simulink model "CH9_1_firstEV_00"  (R2022a)
settings: Solver=VariableStepAuto  StartTime=0.0  StopTime=200  RelTol=1e-3
values from neighbouring files (symbols this model uses):
  Batt_R0 = 0.05    [CH9_1_firstEV_00Param.m]    (also in CH9_1_firstEV_01Param.m; CH9_1_firstEV_02Param.m)
  Motor_kTorque = 0.01    [CH9_1_firstEV_00Param.m]    (also in CH9_1_firstEV_01Param.m; CH9_1_firstEV_02Param.m)
  Motor_TrqKi = 400    [CH9_1_firstEV_00Param.m]    (also in CH9_1_firstEV_01Param.m; CH9_1_firstEV_02Param.m)
  Motor_TrqKp = 600    [CH9_1_firstEV_00Param.m]    (also in CH9_1_firstEV_01Param.m; CH9_1_firstEV_02Param.m)
  Motor_TrqMax = 400    [CH9_1_firstEV_00Param.m]    (also in CH9_1_firstEV_01Param.m; CH9_1_firstEV_02Param.m)
  Motor_TrqMin = -400    [CH9_1_firstEV_00Param.m]    (also in CH9_1_firstEV_01Param.m; CH9_1_firstEV_02Param.m)
  Motor_tTorque = 0.02    [CH9_1_firstEV_00Param.m]    (also in CH9_1_firstEV_01Param.m; CH9_1_firstEV_02Param.m)
  VehMass = 1200    [CH9_1_firstEV_00Param.m]    (also in CH9_1_firstEV_01Param.m)
libraries: fl_lib x34, nesl_utility x9, sdl_lib x6, autolibshared x1, ee_lib x1, slpidlib x1
settings Model: Creator=amyyang  LastModifiedBy=amyyang
settings SolverCC: ZeroCrossAlgorithm=Adaptive  AlgebraicLoopSolver=TrustRegion
settings DataIOCC: ReturnWorkspaceOutputs=off
settings DebuggingCC: IgnoredZcDiagnostic=none  UnconnectedInputMsg=warning  UnconnectedOutputMsg=warning  UnconnectedLineMsg=warning  SFMachineParentedDataDiag=warning  ArithmeticOperatorsInVariantConditions=warning
settings SFSimCC: SimUseLocalCustomCode=off  CustomCodeUndefinedFunction=UseInterfaceOnly
settings RTWCC: RTWUseLocalCustomCode=off  DLArmComputeVersion=19.05
settings SimscapeCC: SimscapeLogType=local  SimscapeLogSimulationStatistics=on  SimscapeLogToSDI=on  SimscapeLogLimitData=off

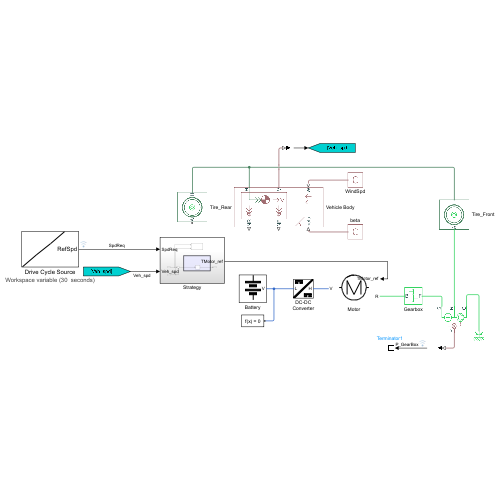
[thumbnail: Simulink's stored preview of the top-level diagram]
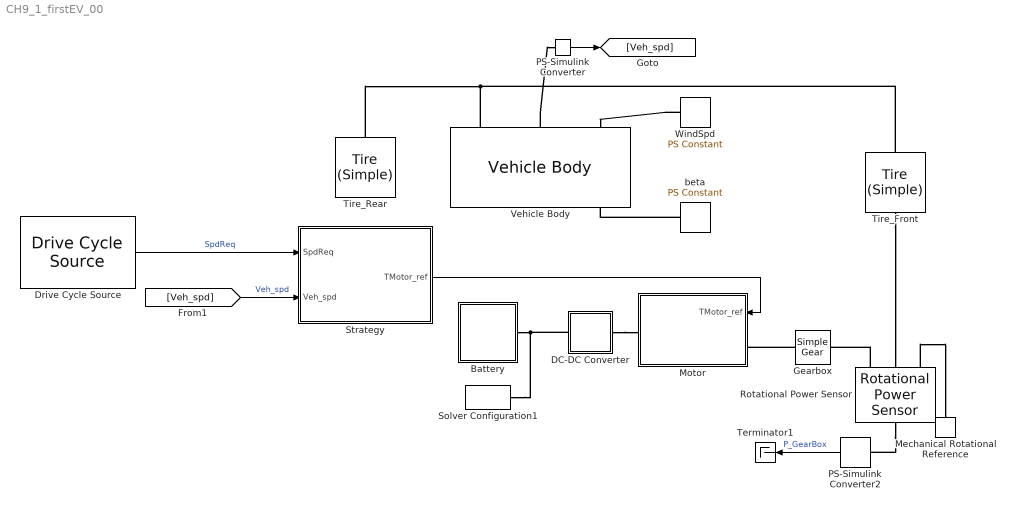
== system CH9_1_firstEV_00 ==
  Battery : Subsystem
      mask Display:
      | % Plot points to set plot range
      | color('white');plot(1.5, 2.5);plot(-1.5, -2)
      | color('black');
      | % Battery icon
      | plot([0 0], [2.5 1.3])
      | plot([0 0], [-0.6 -1.6])
      | patch([-1 1 1 -1]*0.4, [1 1 -1 -1]*0.15+0.7,[0;0;0]);
      | patch([-1 1 1 -1]*0.4, [1 1 -1 -1]*0.15-0.6,[0;0;0]);
      | patch([-1 1 1 -1]*0.8, [1 1 -1 -1]*0.15+1.3,[0;0;0]);
      | patch([-1 1 1 -1]*0.8, [1 1 -1 -1]*0.15+0.0,[0;0;0]);
  DC-DC Converter : Subsystem
      mask Display:
      | patch([-0.9 -1 -1 0.9 1 1 -0.9],[-1 -1 -0.9 1 1 0.9 -1],[0 0 0])
      | 
      | patch([-0.8 -0.1 -0.1 -0.8],[0.85 0.85 0.75 0.75],[0 0 0])
      | patch([-0.8 -0.55 -0.55 -0.8],[0.65 0.65 0.55 0.55],[0 0 0])
      | patch([-0.35 -0.1 -0.1 -0.35],[0.65 0.65 0.55 0.55],[0 0 0])
      | 
      | patch([-0.8 -0.1 -0.1 -0.8]*-1,[0.65 0.65 0.55 0.55]*-1,[0 0 0])
      | patch([-0.8 -0.55 -0.55 -0.8]*-1,[0.85 0.85 0.75 0.75]*-1,[0 0 0])
      | patch([-0.35 -0.1 -0.1 -0.35]*-1,[0.85 0.85 0.75 0.75]*-1,[0 0 0])
  Drive Cycle Source : autolibshared/Drive Cycle Source  cycleVar=Workspace variable  wsVar=myCycleS  fileVar=cycleFTP75.mat  tfinal="30  seconds"  cycleRepeat=off  outAccPort=off  outGearPort=off  gearList=No gear data  t_wot1=5  xdot_woto=0  xdot_wot1=30  t_wot2=20  xdot_wot2=0  t_wotend=30  srcUnit=m/s  outUnit=m/s  srcAccUnit=m/s/s  outAccUnit=m/s^2  dt=0  aMode=1  faultOption=off  velBnd=2  velBndUnit=mph  inUnit=m/s  timeBnd=1  failOption=off  stopSim=off  maxFaultCnt=10  maxFaultTime=2  maxTotFaultTime=15  traceOption=off  dtTrace=1  traceWindow=10  lastDCname=Custom Data Set  lastOutUnit=mph  lastDT=0  lastTB=1  lastSB=2  forceCalcBound=off
      settings: SourceProductBaseCode=PW,DR,MT,VE
  Gearbox : sdl_lib/Gears/Simple Gear  ratio=Motor_GearRio  rotation_direction=sdl.enum.shaftOutputDirection.same  friction_model=sdl.enum.gear_efficiencies_load.constant  T_noload=0.1 N*m  T_nom=5 N*m  efficiency_nom=0.8  efficiency=Motor_GearEff  temperature_TLU=[ 280 300 320 ] K  load_TLU=[ 1 5 10 ] N*m  efficiency_TLU=[ 0.95 0.9 0.85 ]  efficiency_TLU2=[ 0.85 0.8 0.75; 0.95 0.9 0.85; 0.85 0.8 0.7 ]  w_thr=0.01 rad/s  pwr_thr=0.001 W  backlash_model=sdl.enum.backlashModel.Off  backlash_distance=1e-3 mm  x0=0 mm  r_base=0.1 m  hardstop_model=simscape.enum.hardstop.smooth  transition=1e-4 mm  backlash_stiffness=1e7 N/m  backlash_damping=1e6 N*s/m  e=0  v_tol=0.001 m/s  mu_visc=[ 0 0 ] N*m/(rad/s)  enable_faults=simscape.enum.onoff.off  efficiency_fault=0.05  external_fault=simscape.enum.onoff.off  temporal_fault=simscape.enum.onoff.off  fault_time=5 s  fault_angles=pi / 12 rad  report_fault=simscape.enum.assert.action.none  thermal_mass=50 J/K  temperature_specify=off  temperature_priority=High  temperature=300 K  temperature_nominal_specify=off  temperature_nominal_unit=K  temperature_nominal_value=1  x_backlash_specify=off  x_backlash_priority=None  x_backlash=0 mm  x_backlash_nominal_specify=off  x_backlash_nominal_unit=mm  x_backlash_nominal_value=1  f_hardstop_specify=off  f_hardstop_priority=None  f_hardstop=0 N  f_hardstop_nominal_specify=off  f_hardstop_nominal_unit=N  f_hardstop_nominal_value=1  v_backlash_specify=off  v_backlash_priority=None  v_backlash=0 m/s  v_backlash_nominal_specify=off  v_backlash_nominal_unit=m/s  v_backlash_nominal_value=1
      settings: SourceProductName=Driveline  LogSimulationData=on
  Mechanical Rotational Reference : fl_lib/Mechanical/Rotational Elements/Mechanical Rotational Reference
      settings: SourceProductBaseCode=PW,SS,VE
  Motor : Subsystem
      mask Display:
      | % Circle
      | plot(sin(0:0.1:2.2*pi)*0.9,cos(0:0.1:2.2*pi)*0.9);
      | 
      | % In/out
      | plot([-1.1 -0.9],[0 0]);
      | plot([1.1 0.9],[0 0]);
      | 
      | % 'M'
      | plot([0.5 0.5],[-0.5 0.5]);
      | plot([-0.5 -0.5],[-0.5 0.5]);
      | plot([0.5 0],[0.5 -0.5]);
      | plot([-0.5 0],[0.5 -0.5]);
      | 
      | % Plot points to set plot range
      | color('white');plot(1.9,1.2);plot(-1.9,-1.2)
      | color('black');
  PS-Simulink Converter : nesl_utility/PS-Simulink Converter  PhysicalDomain=network_engine_domain  SubClassName=ps_output  LeftPortType=input  RightPortType=output  PseudoPeriodic=off  Frequencies=[]  VectorFormat=1-D array  Unit=m/s  AffineConversion=off
      settings: SourceProductBaseCode=SS,PW,VE
  PS-Simulink Converter2 : nesl_utility/PS-Simulink Converter  PhysicalDomain=network_engine_domain  SubClassName=ps_output  LeftPortType=input  RightPortType=output  PseudoPeriodic=off  Frequencies=[]  VectorFormat=1-D array  Unit=kW  AffineConversion=off
      settings: SourceProductName=Utilities
  Rotational Power Sensor : sdl_lib/Sensors/Rotational Power Sensor  measurement_type=1  averaging_period=1 s  max_frequency=1000 Hz  max_speed=1000 rpm
      settings: SourceProductBaseCode=LD  InternalSimscapePortConfiguration="{\"Bottom\":[],\"Left\":[{\"id\":\"S\",\"label\":\"S\",\"type\":\"foundation.mechanical.rotational.rotational\"},{\"id\":\"R\",\"label\":\"R\",\"type\":\"foundation.mechanical.rotational.rotational\"},{\"id\":\"C\",\"label\":\"C\",\"type\":\"foundation.mechanical.rotational.rotational\"}],\"Right\":[{\"id\":\"P\",\"label\":\"P\",\"type\":\"output\"}],\"Top\":[]}"
  Solver Configuration1 : nesl_utility/Solver Configuration  PhysicalDomain=network_engine_domain  SubClassName=solver  LeftPortType=input  RightPortType=generic  Tones=[]  Harmonics=[]  SimulateNoise=off  Profile=off  UseLocalSampling=off  EnableSwitchedLinearOptims=on  FrequencyDomain=off  UseCCode=off  RelTol=0.001  AbsTol=1e-06  MinStep=1e-09  ToWorkspace=off  RevertToSquareIcSolve=off  NumHomotopyIterations=100  PhasorMode=off  PhasorModeNumHarmonics=1  IndexReductionMethod=DerivativeReplacement  DoDC=off  ResidualTolerance=1e-9  UseLocalSolver=off  LocalSolverChoice=NE_PARTITIONING_ADVANCER  LocalSolverSampleTime=0.005  DoFixedCost=off  MaxNonlinIter=5  MaxModeIter=2  ComputeImpulses=off  ImpulseIterations=2  LinearAlgebra=auto  LinearAlgebraNumThread=0  EquationFormulation=NE_TIME_EF  DelaysMemoryBudget=1024  AutomaticFiltering=on  FilteringTimeConstant=0.001  PartitionStorageMethod=EXHAUSTIVE  PartitionMemoryBudget=1024  PartitionMethod=ROBUST
      settings: SourceProductName=Utilities
  Strategy : Subsystem
  Terminator1 : Terminator
  Tire_Front : sdl_lib/Tires & Vehicles/Tire (Simple)  r_tire=Tire_R m  model_compliance=0  stiffness=Tire_K N/m  damping=Tire_Damp N/(m/s)  model_inertia=0  tire_inertia=Tire_Inertia kg*m^2  initial_velocity=Tire_IniSpd rad/s
      settings: SourceProductBaseCode=LD  LogSimulationData=on  InternalSimscapePortConfiguration="{\"Bottom\":[],\"Left\":[{\"id\":\"A\",\"label\":\"A\",\"type\":\"foundation.mechanical.rotational.rotational\"}],\"Right\":[{\"id\":\"H\",\"label\":\"H\",\"type\":\"foundation.mechanical.translational.translational\"}],\"Top\":[]}"
  Tire_Rear : sdl_lib/Tires & Vehicles/Tire (Simple)  r_tire=Tire_R m  model_compliance=0  stiffness=Tire_K N/m  damping=Tire_Damp N/(m/s)  model_inertia=0  tire_inertia=Tire_Inertia kg*m^2  initial_velocity=Tire_IniSpd rad/s
      settings: SourceProductBaseCode=LD  LogSimulationData=on  InternalSimscapePortConfiguration="{\"Bottom\":[],\"Left\":[{\"id\":\"A\",\"label\":\"A\",\"type\":\"foundation.mechanical.rotational.rotational\"}],\"Right\":[{\"id\":\"H\",\"label\":\"H\",\"type\":\"foundation.mechanical.translational.translational\"}],\"Top\":[]}"
  Vehicle Body : sdl_lib/Tires & Vehicles/Vehicle Body  mass=VehMass kg  n_w=VehWhlperAxle  x_f=VehFrontDis m  x_r=VehRearDis m  y_c=VehCGhight m  mass_var=simscape.enum.onoff.off  g=9.81 m/s^2  liftoff_warning=simscape.enum.onoff.off  area=VehFrontalA m^2  Cd=VehDragCoeff  rho=AirDensity kg/m^3  model_pitch=simscape.enum.onoff.off  inertia=4000 kg*m^2  suspension_model=sdl.enum.linearTLU.linear  k_f=1e4 N/m  b_f=1e4 N/(m/s)  k_r=1e4 N/m  b_r=1e4 N/(m/s)  k_f_TLU=[-2000, -1000, 0, 1000, 2000] N  x_f_TLU=[-.4, -.2, 0, .2, .4] m  b_f_TLU=[-200, -100, 0, 100, 200] N  v_f_TLU=[-4, -2, 0, 2, 4] m/s  k_r_TLU=[-2000, -1000, 0, 1000, 2000] N  x_r_TLU=[-.4, -.2, 0, .2, .4] m  b_r_TLU=[-200, -100, 0, 100, 200] N  v_r_TLU=[-4, -2, 0, 2, 4] m/s  interp_method=simscape.enum.interpolation.linear  extrap_method=simscape.enum.extrapolation.linear  model_hardstop=simscape.enum.onoff.off  upper_bound_f=.25 m  lower_bound_f=-.25 m  stop_k_f=1e6 N/m  stop_b_f=150 N/(m/s)  upper_bound_r=.25 m  lower_bound_r=-.25 m  stop_k_r=1e6 N/m  stop_b_r=150 N/(m/s)  initial_pitch=0 rad  initial_pitch_rate=0 rad/s  v_specify=on  v_priority=High  v=Veh_SpdIni m/s  v_nominal_specify=off  v_nominal_unit=m/s  v_nominal_value=1
      settings: LogSimulationData=on
  WindSpd : fl_lib/Physical Signals/Sources/PS Constant  constant=windSpd m/s
      settings: SourceProductBaseCode=PW,SS,VE
  beta : fl_lib/Physical Signals/Sources/PS Constant  constant=0
      settings: SourceProductBaseCode=PW,SS,VE
  wires:
  Drive Cycle Source/1 -> Strategy/1(SpdReq)  "SpdReq"
  Strategy/1(TMotor_ref) -> Motor/1(TMotor_ref)
  PS-Simulink Converter/1 -> [Veh_spd]
  [Veh_spd] -> Strategy/2(Veh_spd)  "Veh_spd"
  PS-Simulink Converter2/1 -> Terminator1/1  "P_GearBox"
  connections:
  Vehicle Body/LConn1 -- Tire_Rear/RConn1 -- Tire_Front/RConn1
  beta/RConn1 -- Vehicle Body/RConn3
  WindSpd/RConn1 -- Vehicle Body/LConn3
  Solver Configuration1/RConn1 -- DC-DC Converter/LConn1 -- Battery/LConn1
  DC-DC Converter/RConn1 -- Motor/RConn1
  Vehicle Body/LConn2 -- PS-Simulink Converter/LConn1
  Rotational Power Sensor/RConn1 -- PS-Simulink Converter2/LConn1
  Rotational Power Sensor/LConn3 -- Mechanical Rotational Reference/LConn1
  Gearbox/LConn1 -- Motor/LConn1
  Rotational Power Sensor/LConn1 -- Gearbox/RConn1
  Tire_Front/LConn1 -- Rotational Power Sensor/LConn2

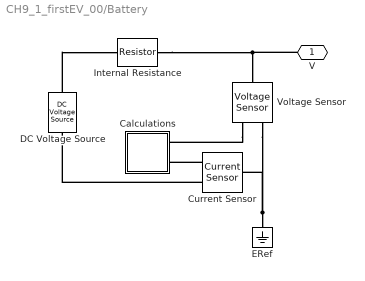
== system CH9_1_firstEV_00/Battery ==
  Calculations : Subsystem
  Current Sensor : fl_lib/Electrical/Electrical Sensors/Current Sensor
      settings: SourceProductName=Foundation Library
  DC Voltage Source : fl_lib/Electrical/Electrical Sources/DC Voltage Source  v0=Batt_V V
      settings: SourceProductName=Foundation Library
  ERef : fl_lib/Electrical/Electrical Elements/Electrical Reference
      settings: SourceProductName=Foundation Library
  Internal Resistance : fl_lib/Electrical/Electrical Elements/Resistor  R=Batt_R0 Ohm  i_specify=off  i_priority=High  i=0 A  i_nominal_specify=off  i_nominal_unit=A  i_nominal_value=1  v_specify=off  v_priority=High  v=0 V  v_nominal_specify=off  v_nominal_unit=V  v_nominal_value=1
      settings: SourceProductName=Foundation Library
  Voltage Sensor : fl_lib/Electrical/Electrical Sensors/Voltage Sensor
      settings: SourceProductName=Foundation Library
  V : PMIOPort  Side=Left
  connections:
  DC Voltage Source/LConn1 -- Internal Resistance/LConn1
  Internal Resistance/RConn1 -- V/RConn1 -- Voltage Sensor/LConn1
  Current Sensor/RConn2 -- DC Voltage Source/RConn1
  Voltage Sensor/RConn1 -- Calculations/LConn1
  Current Sensor/RConn1 -- Calculations/LConn2
  ERef/LConn1 -- Current Sensor/LConn1 -- Voltage Sensor/RConn2

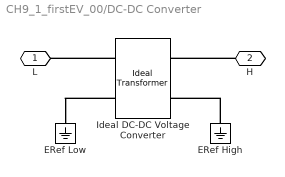
== system CH9_1_firstEV_00/DC-DC Converter ==
  ERef High : fl_lib/Electrical/Electrical Elements/Electrical Reference
      settings: SourceProductName=Foundation Library
  ERef Low : fl_lib/Electrical/Electrical Elements/Electrical Reference
      settings: SourceProductName=Foundation Library
  Ideal DC-DC Voltage Converter : fl_lib/Electrical/Electrical Elements/Ideal Transformer  n=DCDC_WindingRio  i1_specify=off  i1_priority=None  i1=0 A  i1_nominal_specify=off  i1_nominal_unit=A  i1_nominal_value=1  v1_specify=off  v1_priority=None  v1=0 V  v1_nominal_specify=off  v1_nominal_unit=V  v1_nominal_value=1  i2_specify=off  i2_priority=None  i2=0 A  i2_nominal_specify=off  i2_nominal_unit=A  i2_nominal_value=1  v2_specify=off  v2_priority=None  v2=0 V  v2_nominal_specify=off  v2_nominal_unit=V  v2_nominal_value=1
      settings: SourceProductName=Foundation Library
  L : PMIOPort  Tag=PMCPort  Side=Left
  H : PMIOPort  Port=2  Side=Right
  connections:
  ERef High/LConn1 -- Ideal DC-DC Voltage Converter/RConn2
  H/RConn1 -- Ideal DC-DC Voltage Converter/RConn1
  Ideal DC-DC Voltage Converter/LConn2 -- ERef Low/LConn1
  Ideal DC-DC Voltage Converter/LConn1 -- L/RConn1

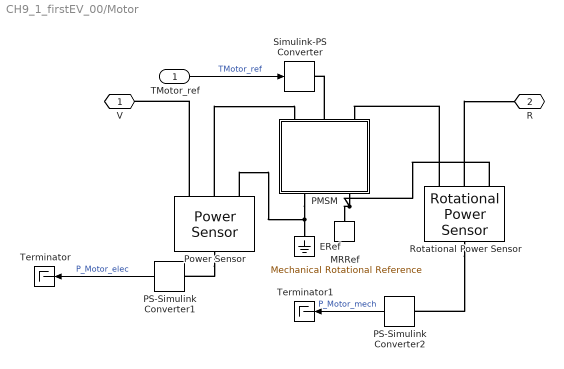
== system CH9_1_firstEV_00/Motor ==
  TMotor_ref : Inport
  ERef : fl_lib/Electrical/Electrical Elements/Electrical Reference
      settings: SourceProductName=Foundation Library
  MRRef : fl_lib/Mechanical/Rotational Elements/Mechanical Rotational Reference
      settings: SourceProductName=Foundation Library
  PMSM : Subsystem
  PS-Simulink Converter1 : nesl_utility/PS-Simulink Converter  PhysicalDomain=network_engine_domain  SubClassName=ps_output  LeftPortType=input  RightPortType=output  PseudoPeriodic=off  Frequencies=[]  VectorFormat=1-D array  Unit=kW  AffineConversion=off
      settings: SourceProductName=Utilities
  PS-Simulink Converter2 : nesl_utility/PS-Simulink Converter  PhysicalDomain=network_engine_domain  SubClassName=ps_output  LeftPortType=input  RightPortType=output  PseudoPeriodic=off  Frequencies=[]  VectorFormat=1-D array  Unit=kW  AffineConversion=off
      settings: SourceProductName=Utilities
  Power Sensor : ee_lib/Sensors & Transducers/Power Sensor  measurement_type=1  averaging_period=1e-4 s
      settings: SourceProductBaseCode=PS
  Rotational Power Sensor : sdl_lib/Sensors/Rotational Power Sensor  measurement_type=1  averaging_period=1 s  max_frequency=1000 Hz  max_speed=1000 rpm
      settings: SourceProductBaseCode=LD  InternalSimscapePortConfiguration="{\"Bottom\":[],\"Left\":[{\"id\":\"S\",\"label\":\"S\",\"type\":\"foundation.mechanical.rotational.rotational\"},{\"id\":\"R\",\"label\":\"R\",\"type\":\"foundation.mechanical.rotational.rotational\"},{\"id\":\"C\",\"label\":\"C\",\"type\":\"foundation.mechanical.rotational.rotational\"}],\"Right\":[{\"id\":\"P\",\"label\":\"P\",\"type\":\"output\"}],\"Top\":[]}"
  Simulink-PS Converter : nesl_utility/Simulink-PS Converter  PhysicalDomain=network_engine_domain  SubClassName=ps_input  LeftPortType=input  RightPortType=output  PseudoPeriodic=off  Frequencies=[]  NoiseDistribution=none  NoiseParameters=[]  Unit=N*m  AffineConversion=off  FilteringAndDerivatives=zero  SimscapeFilterOrder=1  InputFilterTimeConstant=.001  UdotUserProvided=0
      settings: SourceProductName=Utilities
  Terminator : Terminator
  Terminator1 : Terminator
  V : PMIOPort  Side=Right
  R : PMIOPort  Port=2  Side=Left
  wires:
  TMotor_ref/1 -> Simulink-PS Converter/1  "TMotor_ref"
  PS-Simulink Converter1/1 -> Terminator/1  "P_Motor_elec"
  PS-Simulink Converter2/1 -> Terminator1/1  "P_Motor_mech"
  connections:
  PMSM/RConn1 -- Power Sensor/LConn3 -- ERef/LConn1
  PMSM/RConn2 -- Rotational Power Sensor/LConn3 -- MRRef/LConn1
  PMSM/LConn2 -- Simulink-PS Converter/RConn1
  Power Sensor/RConn1 -- PS-Simulink Converter1/LConn1
  Power Sensor/LConn1 -- V/RConn1
  Power Sensor/LConn2 -- PMSM/LConn1
  Rotational Power Sensor/RConn1 -- PS-Simulink Converter2/LConn1
  Rotational Power Sensor/LConn1 -- PMSM/LConn3
  Rotational Power Sensor/LConn2 -- R/RConn1

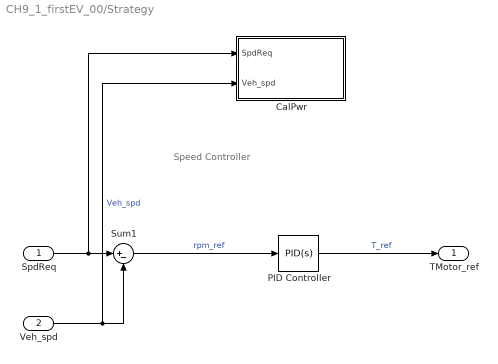
== system CH9_1_firstEV_00/Strategy ==
  note: Speed
      | Controller
  SpdReq : Inport
  Veh_spd : Inport  Port=2
  CalPwr : Subsystem
  PID Controller : slpidlib/PID Controller  Controller=PID  Form=Parallel  TimeDomain=Continuous-time  UseExternalTs=off  SampleTime=-1  IntegratorMethod=Forward Euler  FilterMethod=Forward Euler  ControllerParametersSource=internal  P=Motor_TrqKp  I=Motor_TrqKi  UseKiTs=off  D=0.039394783828742  N=0.280588301881495  UseFilter=on  TunerSelectOption=Transfer Function Based (PID Tuner App)  InitialConditionSource=internal  InitialConditionForIntegrator=0  InitialConditionForFilter=0  DifferentiatorICPrevScaledInput=0  ExternalReset=none  TrackingMode=off  Kt=1  LimitOutput=on  SatLimitsSource=internal  UpperSaturationLimit=Motor_TrqMax  LowerSaturationLimit=Motor_TrqMin  LinearizeAsGain=on  AntiWindupMode=none  Kb=1  POutMin=[]  POutMax=[]  IOutMin=[]  IOutMax=[]  DOutMin=[]  DOutMax=[]  NOutMin=[]  NOutMax=[]  SumOutMin=[]  SumOutMax=[]  SaturationOutMin=[]  SaturationOutMax=[]  PParamMin=[]  PParamMax=[]  IParamMin=[]  IParamMax=[]  DParamMin=[]  DParamMax=[]  NParamMin=[]  NParamMax=[]  KbParamMin=[]  KbParamMax=[]  KtParamMin=[]  KtParamMax=[]  KbOutMin=[]  KbOutMax=[]  KtOutMin=[]  KtOutMax=[]  IntegratorOutMin=[]  IntegratorOutMax=[]  FilterOutMin=[]  FilterOutMax=[]  SumI1OutMin=[]  SumI1OutMax=[]  SumI2OutMin=[]  SumI2OutMax=[]  SumI3OutMin=[]  SumI3OutMax=[]  SumI4OutMin=[]  SumI4OutMax=[]  SumDOutMin=[]  SumDOutMax=[]  DifferentiatorOutMin=[]  DifferentiatorOutMax=[]  FilterDiffOutCoefMin=[]  FilterDiffOutCoefMax=[]  ReciprocalOutMin=[]  ReciprocalOutMax=[]  SumDenOutMin=[]  SumDenOutMax=[]  SumNumOutMin=[]  SumNumOutMax=[]  DivideOutMin=[]  DivideOutMax=[]  UdiffTsProdOutMin=[]  UdiffTsProdOutMax=[]  NTsProdOutMin=[]  NTsProdOutMax=[]  UintegralTsProdOutMin=[]  UintegralTsProdOutMax=[]  UngainTsProdOutMin=[]  UngainTsProdOutMax=[]  IntegratorContinuousStateAttributes=''  IntegratorStateMustResolveToSignalObject=off  IntegratorRTWStateStorageClass=Auto  FilterContinuousStateAttributes=''  FilterStateMustResolveToSignalObject=off  FilterRTWStateStorageClass=Auto  ParallelPVariant=InternalParameters  IdealPVariant=Disabled  IVariant=InternalParameters  DVariant=InternalParameters  IntegratorVariant=Continuous  SatVariant=Enabled  AWVariant=Passthrough  PCopyVariant=Disabled  TRVariant=Disabled  FdbkBlocksVariant=Forward  IdealPFdbkVariant=Disabled  SatFdbkVariant=Disabled  DerivativeFilterVariant=ContFilter  NVariant=InternalParameters  NCopyVariant=Disabled  FilterICVariant=InternalICsFilter  IntegratorICVariant=InternalICs  ExternalResetVariant=Disabled  TRSumVariant=Passthrough  SumFdbkVariant=Disabled  SumVariant=Sum_PID  TsampFilterVariant=InternalTs  TsampNgainVariant=Passthrough  TsampIntegralVariant=Passthrough  ExternalSaturationOutDataTypeStr=Inherit: Same as second input  aMode=0
  Sum1 : Sum  Inputs=|+-
  TMotor_ref : Outport
  wires:
  Veh_spd/1 -> CalPwr/2(Veh_spd), Sum1/2  "Veh_spd"
  PID Controller/1 -> TMotor_ref/1  "T_ref"
  Sum1/1 -> PID Controller/1  "rpm_ref"
  SpdReq/1 -> CalPwr/1(SpdReq), Sum1/1

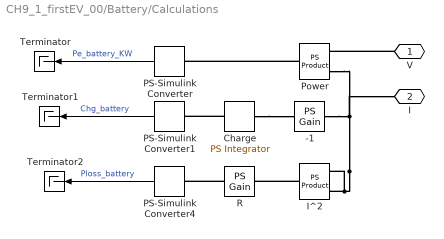
== system CH9_1_firstEV_00/Battery/Calculations ==
  -1 : fl_lib/Physical Signals/Functions/PS Gain  gain=-1
      settings: SourceProductBaseCode=PW,SS,VE
  Charge : fl_lib/Physical Signals/Linear Operators/PS Integrator  reset_method=foundation.enum.IntegratorResetSpec.None  initial_condition_spec=foundation.enum.IntegratorICSpec.Internal  x0=150 A*hr
      settings: SourceProductName=Foundation Library
  I^2 : fl_lib/Physical Signals/Functions/PS Product
      settings: SourceProductName=Foundation Library
  PS-Simulink Converter : nesl_utility/PS-Simulink Converter  PhysicalDomain=network_engine_domain  SubClassName=ps_output  LeftPortType=input  RightPortType=output  PseudoPeriodic=off  Frequencies=[]  VectorFormat=1-D array  Unit=kW  AffineConversion=off
      settings: SourceProductName=Utilities
  PS-Simulink Converter1 : nesl_utility/PS-Simulink Converter  PhysicalDomain=network_engine_domain  SubClassName=ps_output  LeftPortType=input  RightPortType=output  PseudoPeriodic=off  Frequencies=[]  VectorFormat=1-D array  Unit=A*hr  AffineConversion=off
      settings: SourceProductName=Utilities
  PS-Simulink Converter4 : nesl_utility/PS-Simulink Converter  PhysicalDomain=network_engine_domain  SubClassName=ps_output  LeftPortType=input  RightPortType=output  PseudoPeriodic=off  Frequencies=[]  VectorFormat=1-D array  Unit=kW  AffineConversion=off
      settings: SourceProductName=Utilities
  Power : fl_lib/Physical Signals/Functions/PS Product
      settings: SourceProductName=Foundation Library
  R : fl_lib/Physical Signals/Functions/PS Gain  gain=Batt_R0 V/A
      settings: SourceProductName=Foundation Library
  Terminator : Terminator
  Terminator1 : Terminator
  Terminator2 : Terminator
  V : PMIOPort  Side=Left
  I : PMIOPort  Port=2  Side=Left
  wires:
  PS-Simulink Converter4/1 -> Terminator2/1  "Ploss_battery"
  PS-Simulink Converter1/1 -> Terminator1/1  "Chg_battery"
  PS-Simulink Converter/1 -> Terminator/1  "Pe_battery_KW"
  connections:
  R/RConn1 -- PS-Simulink Converter4/LConn1
  I^2/RConn1 -- R/LConn1
  I^2/LConn2 -- -1/LConn1 -- I/RConn1 -- Power/LConn2 -- I^2/LConn1
  V/RConn1 -- Power/LConn1
  Power/RConn1 -- PS-Simulink Converter/LConn1
  Charge/RConn1 -- PS-Simulink Converter1/LConn1
  Charge/LConn1 -- -1/RConn1

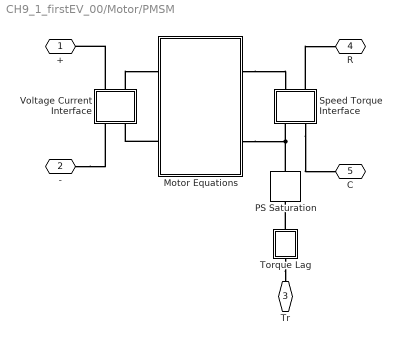
== system CH9_1_firstEV_00/Motor/PMSM ==
  Motor Equations : Subsystem
  PS Saturation : fl_lib/Physical Signals/Nonlinear Operators/PS Saturation  upper_limit=Motor_TrqMax N*m  lower_limit=Motor_TrqMin N*m
      settings: SourceProductBaseCode=PW,SS,VE
  Speed Torque Interface : Subsystem
  Torque Lag : Subsystem
  Voltage Current Interface : Subsystem
  + : PMIOPort  Side=Left
  - : PMIOPort  Port=2  Side=Right
  Tr : PMIOPort  Port=3  Side=Left
  R : PMIOPort  Port=4  Side=Left
  C : PMIOPort  Port=5  Side=Right
  connections:
  Voltage Current Interface/LConn1 -- +/RConn1
  -/RConn1 -- Voltage Current Interface/RConn1
  Speed Torque Interface/LConn2 -- R/RConn1
  Speed Torque Interface/RConn2 -- C/RConn1
  Voltage Current Interface/LConn2 -- Motor Equations/LConn1
  Motor Equations/RConn1 -- Speed Torque Interface/LConn1
  Motor Equations/LConn2 -- Voltage Current Interface/RConn2
  PS Saturation/RConn1 -- Motor Equations/RConn2 -- Speed Torque Interface/RConn1
  Torque Lag/RConn1 -- PS Saturation/LConn1
  Torque Lag/LConn1 -- Tr/RConn1

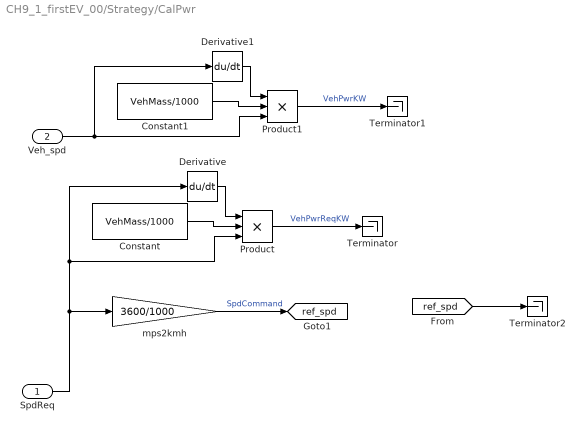
== system CH9_1_firstEV_00/Strategy/CalPwr ==
  SpdReq : Inport  Unit=m/s
  Veh_spd : Inport  Port=2  Unit=m/s
  Constant : Constant  Value=VehMass/1000
  Constant1 : Constant  Value=VehMass/1000
  Derivative : Derivative
  Derivative1 : Derivative
  Product : Product  Inputs=***
  Product1 : Product  Inputs=***
  Terminator : Terminator
  Terminator1 : Terminator
  Terminator2 : Terminator
  mps2kmh : Gain  Gain=3600/1000
  tag scope: ref_spd=global
  wires:
  Product/1 -> Terminator/1  "VehPwrReqKW"
  SpdReq/1 -> mps2kmh/1, Derivative/1, Product/3
  Constant/1 -> Product/2
  Derivative/1 -> Product/1
  mps2kmh/1 -> [ref_spd]  "SpdCommand"
  Derivative1/1 -> Product1/1
  Constant1/1 -> Product1/2
  Veh_spd/1 -> Derivative1/1, Product1/3
  Product1/1 -> Terminator1/1  "VehPwrKW"
  [ref_spd] -> Terminator2/1

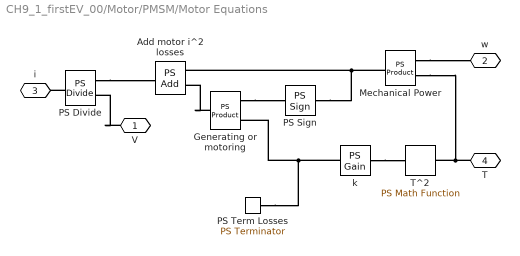
== system CH9_1_firstEV_00/Motor/PMSM/Motor Equations ==
  Add motor i^2 losses : fl_lib/Physical Signals/Functions/PS Add
      settings: SourceProductName=Foundation Library  LogSimulationData=on
  Generating or motoring : fl_lib/Physical Signals/Functions/PS Product
      settings: SourceProductName=Foundation Library
  Mechanical Power : fl_lib/Physical Signals/Functions/PS Product
      settings: SourceProductName=Foundation Library
  PS Divide : fl_lib/Physical Signals/Functions/PS Divide
      settings: SourceProductName=Foundation Library  LogSimulationData=on
  PS Sign : fl_lib/Physical Signals/Nonlinear Operators/PS Sign
      settings: SourceProductName=Foundation Library  InternalSimscapePortConfiguration="{\"Bottom\":[],\"Left\":[{\"id\":\"I\",\"label\":\"\",\"type\":\"input\"}],\"Right\":[{\"id\":\"O\",\"label\":\"\",\"type\":\"output\"}],\"Top\":[]}"
  PS Term Losses : fl_lib/Physical Signals/Sinks/PS Terminator
      settings: SourceProductName=Foundation Library
  T^2 : fl_lib/Physical Signals/Functions/PS Math Function  fcn_choice=7  v=1
      settings: SourceProductName=Foundation Library
  k : fl_lib/Physical Signals/Functions/PS Gain  gain=Motor_kTorque 1/(N*m*s)
      settings: SourceProductName=Foundation Library
  V : PMIOPort  Side=Left
  w : PMIOPort  Port=2  Side=Right
  i : PMIOPort  Port=3  Side=Left
  T : PMIOPort  Port=4  Side=Right
  connections:
  Generating or motoring/LConn1 -- PS Sign/RConn1
  k/LConn1 -- T^2/RConn1
  Mechanical Power/LConn2 -- T/RConn1 -- T^2/LConn1
  Generating or motoring/LConn2 -- k/RConn1 -- PS Term Losses/LConn1
  Mechanical Power/LConn1 -- w/RConn1
  PS Divide/LConn1 -- Add motor i^2 losses/RConn1
  Generating or motoring/RConn1 -- Add motor i^2 losses/LConn2
  PS Sign/LConn1 -- Add motor i^2 losses/LConn1 -- Mechanical Power/RConn1
  PS Divide/RConn1 -- i/RConn1
  V/RConn1 -- PS Divide/LConn2

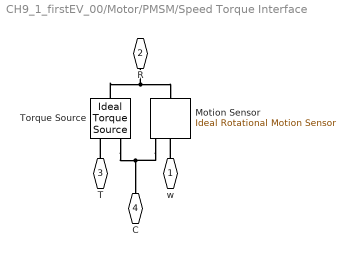
== system CH9_1_firstEV_00/Motor/PMSM/Speed Torque Interface ==
  Motion Sensor : fl_lib/Mechanical/Mechanical Sensors/Ideal Rotational Motion Sensor  wrap_angle=simscape.enum.onoff.off  offset=0 rad
      settings: SourceProductName=Foundation Library
  Torque Source : fl_lib/Mechanical/Mechanical Sources/Ideal Torque Source
      settings: SourceProductName=Foundation Library
  w : PMIOPort  Side=Left
  R : PMIOPort  Port=2  Side=Left
  T : PMIOPort  Port=3  Side=Right
  C : PMIOPort  Port=4  Side=Right
  connections:
  Motion Sensor/RConn1 -- Torque Source/RConn2 -- C/RConn1
  Torque Source/LConn1 -- R/RConn1 -- Motion Sensor/LConn1
  w/RConn1 -- Motion Sensor/RConn2
  T/RConn1 -- Torque Source/RConn1

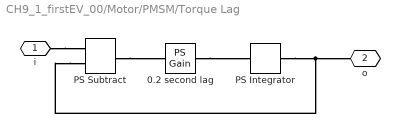
== system CH9_1_firstEV_00/Motor/PMSM/Torque Lag ==
  0.2 second lag : fl_lib/Physical Signals/Functions/PS Gain  gain=1/Motor_tTorque 1/s
      settings: SourceProductName=Foundation Library
  PS Integrator : fl_lib/Physical Signals/Linear Operators/PS Integrator  reset_method=foundation.enum.IntegratorResetSpec.None  initial_condition_spec=foundation.enum.IntegratorICSpec.Internal  x0=0 N*m
      settings: SourceProductName=Foundation Library
  PS Subtract : fl_lib/Physical Signals/Functions/PS Subtract
      settings: SourceProductName=Foundation Library
  i : PMIOPort  Side=Left
  o : PMIOPort  Port=2  Side=Right
  connections:
  i/RConn1 -- PS Subtract/LConn1
  PS Subtract/LConn2 -- o/RConn1 -- PS Integrator/RConn1
  0.2 second lag/RConn1 -- PS Integrator/LConn1
  PS Subtract/RConn1 -- 0.2 second lag/LConn1

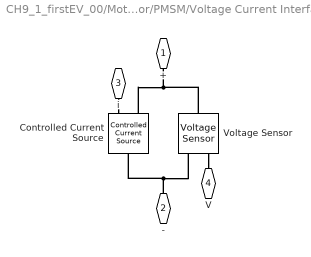
== system CH9_1_firstEV_00/Motor/PMSM/Voltage Current Interface ==
  Controlled Current Source : fl_lib/Electrical/Electrical Sources/Controlled Current Source
      settings: SourceProductName=Foundation Library
  Voltage Sensor : fl_lib/Electrical/Electrical Sensors/Voltage Sensor
      settings: SourceProductName=Foundation Library
  + : PMIOPort  Side=Left
  - : PMIOPort  Port=2  Side=Right
  i : PMIOPort  Port=3  Side=Right
  V : PMIOPort  Port=4  Side=Left
  connections:
  Controlled Current Source/RConn2 -- Voltage Sensor/LConn1 -- +/RConn1
  Voltage Sensor/RConn1 -- V/RConn1
  i/RConn1 -- Controlled Current Source/RConn1
  -/RConn1 -- Controlled Current Source/LConn1 -- Voltage Sensor/RConn2
